simulink model "Encoder_reader_simulink"  (R2025a)
settings: Solver=FixedStepAuto  StartTime=0.0  StopTime=100  FixedStep=0.1  RelTol=1e-3  EnableMultiTasking=on
libraries: stm32f4xxblockslib x8, stm32g4xxblockslib x6
settings Model: STM32="{\"EncoderBlockForG4\":[{\"ID\":\"untitled:1\"},{\"ID\":\"Lab3_Encoder:1\"},{\"ID\":\"Encoder_reader_simulink:1\"},{\"ID\":\"Encoder_reader_simulink:35\"},{\"ID\":\"Encoder_reader_simulink:46\"},{\"ID\":\"Encoder_reader_simulink:93\"},{\"ID\":\"Encoder_reader_simulink:94\"},{\"ID\":\"Encoder_reader_simulink:95\"}],\"DigitalPortRead\":[{\"ID\":\"Encoder_reader_simulink:20\"},{\"ID\":\"Encoder_reader_simulink:21\"},{\"ID\":\"Encoder_reader_simulink:25\"},{\"ID\":\"Encoder_reader_simulink:32\"},{\"ID\":\"Encoder_reader_simulink:43\"},{\"ID\":\"Encoder_reader_simulink:90\"},{\"ID\":\"Encoder_reader_simulink:91\"},{\"ID\":\"Encoder_reader_simulink:92\"}]}"  Creator=User  LastModifiedBy=hp
settings OptimizationCC: DefaultParameterBehavior=Inlined  EnhancedBackFolding=on  PassReuseOutputArgsAs=Individual arguments  ZeroExternalMemoryAtStartup=off  ZeroInternalMemoryAtStartup=off  MaxStackSize=512  OptimizeBlockOrder=speed  DifferentSizesBufferReuse=on  OptimizationCustomize=off  EfficientTunableParamExpr=on
settings DebuggingCC: ParameterTunabilityLossMsg=error
settings HardwareCC: ProdBitPerPointer=32.0  ProdBitPerSizeT=32.0  ProdBitPerPtrDiffT=32.0  ProdLargestAtomicInteger=Long  ProdLargestAtomicFloat=Double  ProdWordSize=32.0  ProdLongLongMode=on  ProdHWDeviceType=ARM Compatible->ARM Cortex-M
settings SFSimCC: MATLABDynamicMemAlloc=off
settings RTWCC: SystemTargetFile=ert.tlc  HardwareBoard=STM32G4xx Based  TemplateMakefile=ert_default_tmf  Toolchain=GNU Tools for ARM Embedded Processors  Description=Embedded Coder
settings CodeAppCC: ForceParamTrailComments=on  IgnoreCustomStorageClasses=off  OperatorAnnotations=on  SimulinkDataObjDesc=on  SFDataObjDesc=on  InsertBlockDesc=on
settings ERTTargetCC: ExtModeTransport=3.0  ExtModeStaticAllocSize=2048.0  TargetLangStandard=C99 (ISO)  CodeReplacementLibrary=ARM Cortex-M  SupportContinuousTime=on

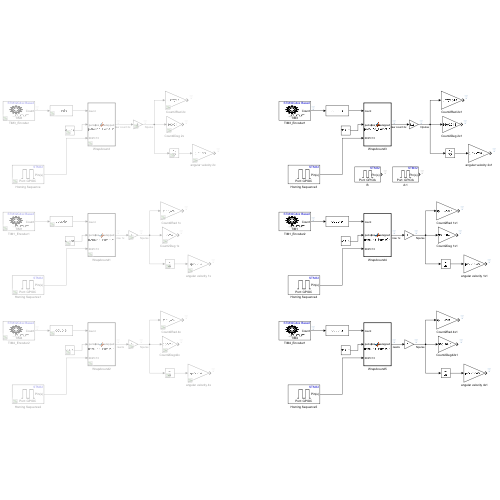
[thumbnail: Simulink's stored preview of the top-level diagram]
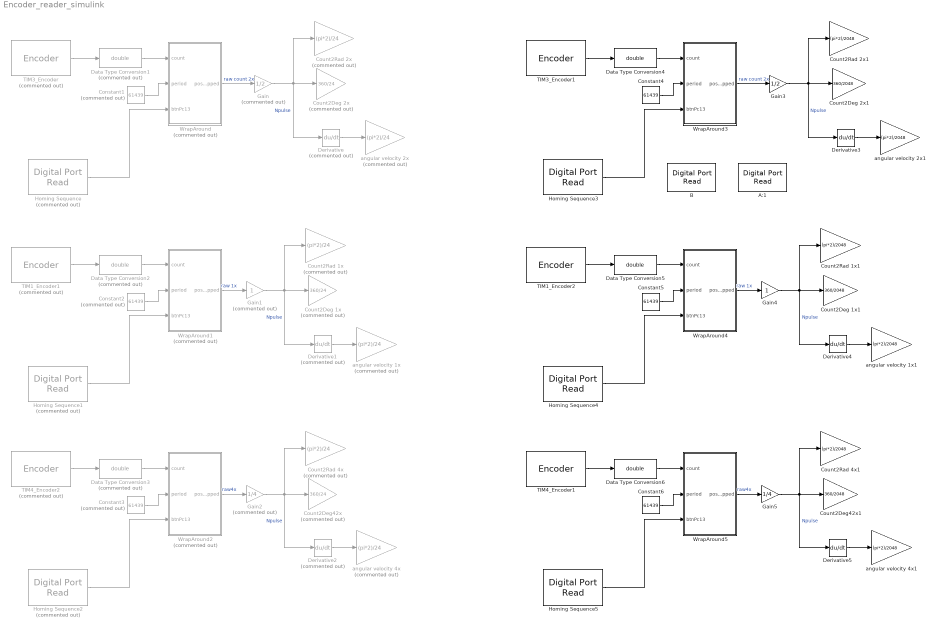
== system Encoder_reader_simulink ==
  A:1 : stm32f4xxblockslib/Digital Port Read  PortName=GPIOA  PinNumber=[4]  ReadOperation=on  IOAsArray=on  SampleTime=-1  EnableSimPort=off  hoistedMaskSrc=ECSoC/ECSimCodegen/Digital Port Read
      settings: LibrarySourceBlock=stm32g4xxblockslib/Digital Port Read
  B : stm32f4xxblockslib/Digital Port Read  PortName=GPIOA  PinNumber=[6]  ReadOperation=on  IOAsArray=on  SampleTime=-1  EnableSimPort=off  hoistedMaskSrc=ECSoC/ECSimCodegen/Digital Port Read
      settings: LibrarySourceBlock=stm32g4xxblockslib/Digital Port Read
  Constant1 : Constant  Commented=on  Value=61439
  Constant2 : Constant  Commented=on  Value=61439
  Constant3 : Constant  Commented=on  Value=61439
  Constant4 : Constant  Value=61439
  Constant5 : Constant  Value=61439
  Constant6 : Constant  Value=61439
  Count2Deg 1x : Gain  Commented=on  Gain=360/24
  Count2Deg 1x1 : Gain  Gain=360/2048
  Count2Deg 2x : Gain  Commented=on  Gain=360/24
  Count2Deg 2x1 : Gain  Gain=360/2048
  Count2Deg42x : Gain  Commented=on  Gain=360/24
  Count2Deg42x1 : Gain  Gain=360/2048
  Count2Rad 1x : Gain  Commented=on  Gain=(pi*2)/24
  Count2Rad 1x1 : Gain  Gain=(pi*2)/2048
  Count2Rad 2x : Gain  Commented=on  Gain=(pi*2)/24
  Count2Rad 2x1 : Gain  Gain=(pi*2)/2048
  Count2Rad 4x : Gain  Commented=on  Gain=(pi*2)/24
  Count2Rad 4x1 : Gain  Gain=(pi*2)/2048
  Data Type Conversion1 : DataTypeConversion  Commented=on  OutDataTypeStr=double  SaturateOnIntegerOverflow=off  RndMeth=Floor
  Data Type Conversion2 : DataTypeConversion  Commented=on  OutDataTypeStr=double  SaturateOnIntegerOverflow=off  RndMeth=Floor
  Data Type Conversion3 : DataTypeConversion  Commented=on  OutDataTypeStr=double  SaturateOnIntegerOverflow=off  RndMeth=Floor
  Data Type Conversion4 : DataTypeConversion  OutDataTypeStr=double  SaturateOnIntegerOverflow=off  RndMeth=Floor
  Data Type Conversion5 : DataTypeConversion  OutDataTypeStr=double  SaturateOnIntegerOverflow=off  RndMeth=Floor
  Data Type Conversion6 : DataTypeConversion  OutDataTypeStr=double  SaturateOnIntegerOverflow=off  RndMeth=Floor
  Derivative : Derivative  Commented=on
  Derivative1 : Derivative  Commented=on
  Derivative2 : Derivative  Commented=on
  Derivative3 : Derivative
  Derivative4 : Derivative
  Derivative5 : Derivative
  Gain : Gain  Commented=on  Gain=1/2
  Gain1 : Gain  Commented=on
  Gain2 : Gain  Commented=on  Gain=1/4
  Gain3 : Gain  Gain=1/2
  Gain4 : Gain
  Gain5 : Gain  Gain=1/4
  Homing Sequence : stm32f4xxblockslib/Digital Port Read  Commented=on  PortName=GPIOC  PinNumber=[13]  ReadOperation=on  IOAsArray=on  SampleTime=-1  EnableSimPort=off  hoistedMaskSrc=ECSoC/ECSimCodegen/Digital Port Read
      settings: LibrarySourceBlock=stm32g4xxblockslib/Digital Port Read
  Homing Sequence1 : stm32f4xxblockslib/Digital Port Read  Commented=on  PortName=GPIOC  PinNumber=[13]  ReadOperation=on  IOAsArray=on  SampleTime=-1  EnableSimPort=off  hoistedMaskSrc=ECSoC/ECSimCodegen/Digital Port Read
      settings: LibrarySourceBlock=stm32g4xxblockslib/Digital Port Read
  Homing Sequence2 : stm32f4xxblockslib/Digital Port Read  Commented=on  PortName=GPIOC  PinNumber=[13]  ReadOperation=on  IOAsArray=on  SampleTime=-1  EnableSimPort=off  hoistedMaskSrc=ECSoC/ECSimCodegen/Digital Port Read
      settings: LibrarySourceBlock=stm32g4xxblockslib/Digital Port Read
  Homing Sequence3 : stm32f4xxblockslib/Digital Port Read  PortName=GPIOC  PinNumber=[13]  ReadOperation=on  IOAsArray=on  SampleTime=-1  EnableSimPort=off  hoistedMaskSrc=ECSoC/ECSimCodegen/Digital Port Read
      settings: LibrarySourceBlock=stm32g4xxblockslib/Digital Port Read
  Homing Sequence4 : stm32f4xxblockslib/Digital Port Read  PortName=GPIOC  PinNumber=[13]  ReadOperation=on  IOAsArray=on  SampleTime=-1  EnableSimPort=off  hoistedMaskSrc=ECSoC/ECSimCodegen/Digital Port Read
      settings: LibrarySourceBlock=stm32g4xxblockslib/Digital Port Read
  Homing Sequence5 : stm32f4xxblockslib/Digital Port Read  PortName=GPIOC  PinNumber=[13]  ReadOperation=on  IOAsArray=on  SampleTime=-1  EnableSimPort=off  hoistedMaskSrc=ECSoC/ECSimCodegen/Digital Port Read
      settings: LibrarySourceBlock=stm32g4xxblockslib/Digital Port Read
  TIM1_Encoder1 : stm32g4xxblockslib/Encoder  Commented=on  TimerModule=TIM1  EnableResetInput=off  OutputCountAfterFirstIndex=off  OutputValidIndex=off  OutputDirection=off  OutputStatus=off  SampleTime=-1
  TIM1_Encoder2 : stm32g4xxblockslib/Encoder  TimerModule=TIM1  EnableResetInput=off  OutputCountAfterFirstIndex=off  OutputValidIndex=off  OutputDirection=off  OutputStatus=off  SampleTime=-1
  TIM3_Encoder : stm32g4xxblockslib/Encoder  Commented=on  TimerModule=TIM3  EnableResetInput=off  OutputCountAfterFirstIndex=off  OutputValidIndex=off  OutputDirection=off  OutputStatus=off  SampleTime=-1
  TIM3_Encoder1 : stm32g4xxblockslib/Encoder  TimerModule=TIM3  EnableResetInput=off  OutputCountAfterFirstIndex=off  OutputValidIndex=off  OutputDirection=off  OutputStatus=off  SampleTime=-1
  TIM4_Encoder1 : stm32g4xxblockslib/Encoder  TimerModule=TIM4  EnableResetInput=off  OutputCountAfterFirstIndex=off  OutputValidIndex=off  OutputDirection=off  OutputStatus=off  SampleTime=-1
  TIM4_Encoder2 : stm32g4xxblockslib/Encoder  Commented=on  TimerModule=TIM4  EnableResetInput=off  OutputCountAfterFirstIndex=off  OutputValidIndex=off  OutputDirection=off  OutputStatus=off  SampleTime=-1
  WrapAround : MATLAB Function  Commented=on  TreatAsAtomicUnit=on
  WrapAround1 : MATLAB Function  Commented=on  TreatAsAtomicUnit=on
  WrapAround2 : MATLAB Function  Commented=on  TreatAsAtomicUnit=on
  WrapAround3 : MATLAB Function  TreatAsAtomicUnit=on
  WrapAround4 : MATLAB Function  TreatAsAtomicUnit=on
  WrapAround5 : MATLAB Function  TreatAsAtomicUnit=on
  angular velocity 1x : Gain  Commented=on  Gain=(pi*2)/24
  angular velocity 1x1 : Gain  Gain=(pi*2)/2048
  angular velocity 2x : Gain  Commented=on  Gain=(pi*2)/24
  angular velocity 2x1 : Gain  Gain=(pi*2)/2048
  angular velocity 4x : Gain  Commented=on  Gain=(pi*2)/24
  angular velocity 4x1 : Gain  Gain=(pi*2)/2048
  wires:
  TIM3_Encoder/1 -> Data Type Conversion1/1
  Data Type Conversion1/1 -> WrapAround/1(count)
  WrapAround/1(pos_unwrapped) -> Gain/1  "raw count 2x"
  Constant1/1 -> WrapAround/2(period)
  Homing Sequence/1 -> WrapAround/3(btnPc13)
  Homing Sequence1/1 -> WrapAround1/3(btnPc13)
  WrapAround1/1(pos_unwrapped) -> Gain1/1  "raw 1x"
  Data Type Conversion2/1 -> WrapAround1/1(count)
  TIM1_Encoder1/1 -> Data Type Conversion2/1
  Constant2/1 -> WrapAround1/2(period)
  Homing Sequence2/1 -> WrapAround2/3(btnPc13)
  WrapAround2/1(pos_unwrapped) -> Gain2/1  "raw4x"
  Data Type Conversion3/1 -> WrapAround2/1(count)
  TIM4_Encoder2/1 -> Data Type Conversion3/1
  Constant3/1 -> WrapAround2/2(period)
  Gain/1 -> Derivative/1, Count2Deg 2x/1, Count2Rad 2x/1  "Npulse"
  Derivative/1 -> angular velocity 2x/1
  Derivative1/1 -> angular velocity 1x/1
  Gain1/1 -> Derivative1/1, Count2Deg 1x/1, Count2Rad 1x/1  "Npulse"
  Gain2/1 -> Derivative2/1, Count2Deg42x/1, Count2Rad 4x/1  "Npulse"
  Derivative2/1 -> angular velocity 4x/1
  WrapAround5/1(pos_unwrapped) -> Gain5/1  "raw4x"
  Derivative5/1 -> angular velocity 4x1/1
  Gain5/1 -> Derivative5/1, Count2Deg42x1/1, Count2Rad 4x1/1  "Npulse"
  Data Type Conversion5/1 -> WrapAround4/1(count)
  Homing Sequence4/1 -> WrapAround4/3(btnPc13)
  TIM1_Encoder2/1 -> Data Type Conversion5/1
  Derivative3/1 -> angular velocity 2x1/1
  Gain3/1 -> Derivative3/1, Count2Deg 2x1/1, Count2Rad 2x1/1  "Npulse"
  Constant6/1 -> WrapAround5/2(period)
  TIM4_Encoder1/1 -> Data Type Conversion6/1
  WrapAround3/1(pos_unwrapped) -> Gain3/1  "raw count 2x"
  Data Type Conversion6/1 -> WrapAround5/1(count)
  Derivative4/1 -> angular velocity 1x1/1
  Homing Sequence3/1 -> WrapAround3/3(btnPc13)
  Data Type Conversion4/1 -> WrapAround3/1(count)
  TIM3_Encoder1/1 -> Data Type Conversion4/1
  Constant5/1 -> WrapAround4/2(period)
  WrapAround4/1(pos_unwrapped) -> Gain4/1  "raw 1x"
  Homing Sequence5/1 -> WrapAround5/3(btnPc13)
  Gain4/1 -> Derivative4/1, Count2Deg 1x1/1, Count2Rad 1x1/1  "Npulse"
  Constant4/1 -> WrapAround3/2(period)

== matlab function Encoder_reader_simulink/WrapAround1 ==
  data: count input; pos_unwrapped output; period input; btnPc13 input
function pos_unwrapped = WrapAround_HomeOnPA5(count, period, btnPc13)
% WrapAround_HomeOnPA5
% - แก้ overflow ของ encoder counter และสะสมตำแหน่งต่อเนื่อง
% - เมื่อ "ปุ่ม PA5" ถูกกด (ขอบขาขึ้นหลังดีบาวน์) ให้รีเซ็ต pos_unwrapped = 0
%
% Inputs
%   count   : ค่าจาก TIMx encoder (0..period)
%   period  : ค่าขอบบนของเคาน์เตอร์ (เช่น 61439) → modulo = period+1
%   btnPc13  : 1 = ปุ่มถูกกด, 0 = ไม่กด (ถ้าเป็น active-low ให้ Invert มาก่อน)
%
% Output
%   pos_unwrapped : ตำแหน่งสะสมแบบต่อเนื่อง (รีเซ็ตเป็น 0 ตอนโฮม)

% ---------- สถานะภายใน ----------
persistent prevCount pos         % สำหรับแก้ wrap และสะสมตำแหน่ง
persistent stableBtn prevStable  % สำหรับดีบาวน์ + ตรวจขอบ
persistent cnt                   % ตัวนับดีบาวน์

if isempty(prevCount)
    prevCount   = double(count);
    pos         = 0.0;
    stableBtn   = false;   % สถานะปุ่มหลังดีบาวน์
    prevStable  = false;   % สถานะปุ่มดีบาวน์ย้อนหลัง 1 สเต็ป
    cnt         = uint16(0);
end

% ---------- แก้ wrap-around ----------
M    = double(period) + 1.0;     % โมดูลัสจริง
half = floor(M/2.0);
d = double(count) - prevCount;
if d >  half
    d = d - M;
elseif d < -half
    d = d + M;
end
pos = pos + d;
prevCount = double(count);

% ---------- ดีบาวน์ปุ่ม (แบบนับตัวอย่างติดกัน) ----------
% ปรับจำนวนตัวอย่างที่ต้องคงที่ก่อนยอมรับการเปลี่ยนสถานะ (N)
N = uint16(5);  % = 5 sample. ถ้า Ts = 1 ms → ~5 ms debounce

raw = (btnPc13 ~= 0);      % ให้เป็น boolean
if raw == stableBtn
    % ไม่มีแนวโน้มเปลี่ยนสถานะ → รีเซ็ตตัวนับ
    cnt = uint16(0);
else
    % มีแนวโน้มเปลี่ยน → นับต่อเนื่องจนถึง N แล้วค่อยสลับสถานะ
    if cnt < N
        cnt = cnt + 1;
    end
    if cnt >= N
        stableBtn = raw;
        cnt = uint16(0);
    end
end

% ---------- ตรวจขอบขาขึ้นหลังดีบาวน์ ----------
rising = (stableBtn == true) && (prevStable == false);
prevStable = stableBtn;

% ---------- รีเซ็ตตำแหน่งเมื่อกด ----------
if rising
    pos = 0.0;     % โฮม: ตั้งค่า pos_unwrapped = 0
end

% ---------- เอาต์พุต ----------
pos_unwrapped = -pos;
end

== matlab function Encoder_reader_simulink/WrapAround ==
  data: count input; pos_unwrapped output; period input; btnPc13 input
function pos_unwrapped=WrapAround_HomeOnPA5(count,period,btnPc13)
%Inputs:
%count   : ค่าจากตัวนับของ TIMx encoder
%period  : ค่าขอบบนของเคาน์เตอร์ (61439) → โมดูลัส = period + 1
%btnPc13 : สัญญาณปุ่ม 1 = กด, 0 = ไม่กด เพื่อ set home
%Output:
%pos_unwrapped : ตำแหน่งสะสมแบบต่อเนื่อง (รีเซ็ตเป็นศูนย์เมื่อโฮม)

persistent prevCount pos
persistent stableBtn prevStable
persistent cnt

if isempty(prevCount)
    % ตรวจว่าฟังก์ชันเพิ่งเริ่มทำงาน (ยังไม่มีค่าเก่า)
    prevCount=double(count);     % ตั้งค่า count เริ่มต้น
    pos=0.0;                     % เริ่มตำแหน่งที่ 0
    stableBtn=false;             % สถานะปุ่มเริ่มต้น = ไม่กด
    prevStable=false;            % สถานะก่อนหน้าเริ่มต้น = ไม่กด
    cnt=uint16(0);               % ตัวนับดีบาวน์เริ่มต้น = 0
end

M=double(period)+1.0;            % โมดูลัสจริงของเคาน์เตอร์ (เช่น 61439+1=61440)
half=floor(M/2.0);               % ครึ่งหนึ่งของโมดูลัส ใช้สำหรับตรวจการ overflow
d=double(count)-prevCount;       % คำนวณความต่างของ count ระหว่างรอบนี้กับรอบก่อน

if d>half
    d=d-M;                       % ถ้าค่ากระโดดบวกมากเกินครึ่ง → ถือว่า wrap จากสูงสุดไปต่ำสุด
elseif d<-half
    d=d+M;                       % ถ้าค่ากระโดดลบมากเกินครึ่ง → ถือว่า wrap จากต่ำสุดไปสูงสุด
end

pos=pos+d;                       % สะสมตำแหน่งแบบต่อเนื่อง (รวมระยะที่เปลี่ยน)
prevCount=double(count);         % เก็บค่า count ปัจจุบันไว้เป็นค่าเดิมสำหรับรอบถัดไป

%---------------- HOMING SEQUENCE ----------------%
N=uint16(5);                     % จำนวน sample ที่ใช้ดีบาวน์ปุ่ม (5 sample → ~5 ms)
raw=(btnPc13~=0);                % อ่านค่าปุ่ม → true ถ้ากด (แปลงเป็น boolean)

if raw==stableBtn
    cnt=uint16(0);               % ถ้าสถานะปุ่มไม่เปลี่ยน → รีเซ็ตตัวนับดีบาวน์
else
    if cnt<N
        cnt=cnt+1;               % ถ้ากำลังเปลี่ยนสถานะ → เพิ่มตัวนับ
    end
    if cnt>=N
        stableBtn=raw;           % ถ้าค่าคงที่ครบ N sample → ยอมรับสถานะใหม่
        cnt=uint16(0);           % รีเซ็ตตัวนับหลังยืนยันสถานะใหม่
    end
end

rising=(stableBtn==true)&&(prevStable==false);
% ตรวจขอบขาขึ้น (จากไม่กด → กด)

prevStable=stableBtn;            % เก็บสถานะปุ่มไว้เป็นค่าก่อนหน้าในรอบถัดไป

if rising
    pos=0.0;                     % ถ้ามีขอบขาขึ้น → รีเซ็ตตำแหน่ง = 0 (Home)
end

pos_unwrapped=-pos;              % สัญญาณเอาต์พุต (กลับขั้วทิศทาง)
end

== matlab function Encoder_reader_simulink/WrapAround2 ==
  data: count input; pos_unwrapped output; period input; btnPc13 input
function pos_unwrapped = WrapAround_HomeOnPA5(count, period, btnPc13)
% WrapAround_HomeOnPA5
% - แก้ overflow ของ encoder counter และสะสมตำแหน่งต่อเนื่อง
% - เมื่อ "ปุ่ม PA5" ถูกกด (ขอบขาขึ้นหลังดีบาวน์) ให้รีเซ็ต pos_unwrapped = 0
%
% Inputs
%   count   : ค่าจาก TIMx encoder (0..period)
%   period  : ค่าขอบบนของเคาน์เตอร์ (เช่น 61439) → modulo = period+1
%   btnPc13  : 1 = ปุ่มถูกกด, 0 = ไม่กด (ถ้าเป็น active-low ให้ Invert มาก่อน)
%
% Output
%   pos_unwrapped : ตำแหน่งสะสมแบบต่อเนื่อง (รีเซ็ตเป็น 0 ตอนโฮม)

% ---------- สถานะภายใน ----------
persistent prevCount pos         % สำหรับแก้ wrap และสะสมตำแหน่ง
persistent stableBtn prevStable  % สำหรับดีบาวน์ + ตรวจขอบ
persistent cnt                   % ตัวนับดีบาวน์

if isempty(prevCount)
    prevCount   = double(count);
    pos         = 0.0;
    stableBtn   = false;   % สถานะปุ่มหลังดีบาวน์
    prevStable  = false;   % สถานะปุ่มดีบาวน์ย้อนหลัง 1 สเต็ป
    cnt         = uint16(0);
end

% ---------- แก้ wrap-around ----------
M    = double(period) + 1.0;     % โมดูลัสจริง
half = floor(M/2.0);
d = double(count) - prevCount;
if d >  half
    d = d - M;
elseif d < -half
    d = d + M;
end
pos = pos + d;
prevCount = double(count);

% ---------- ดีบาวน์ปุ่ม (แบบนับตัวอย่างติดกัน) ----------
% ปรับจำนวนตัวอย่างที่ต้องคงที่ก่อนยอมรับการเปลี่ยนสถานะ (N)
N = uint16(5);  % = 5 sample. ถ้า Ts = 1 ms → ~5 ms debounce

raw = (btnPc13 ~= 0);      % ให้เป็น boolean
if raw == stableBtn
    % ไม่มีแนวโน้มเปลี่ยนสถานะ → รีเซ็ตตัวนับ
    cnt = uint16(0);
else
    % มีแนวโน้มเปลี่ยน → นับต่อเนื่องจนถึง N แล้วค่อยสลับสถานะ
    if cnt < N
        cnt = cnt + 1;
    end
    if cnt >= N
        stableBtn = raw;
        cnt = uint16(0);
    end
end

% ---------- ตรวจขอบขาขึ้นหลังดีบาวน์ ----------
rising = (stableBtn == true) && (prevStable == false);
prevStable = stableBtn;

% ---------- รีเซ็ตตำแหน่งเมื่อกด ----------
if rising
    pos = 0.0;     % โฮม: ตั้งค่า pos_unwrapped = 0
end

% ---------- เอาต์พุต ----------
pos_unwrapped = -pos;
end

== matlab function Encoder_reader_simulink/WrapAround3 ==
  data: count input; pos_unwrapped output; period input; btnPc13 input
function pos_unwrapped = WrapAround_HomeOnPA5(count, period, btnPc13)
persistent prevCount pos         % สำหรับแก้ wrap และสะสมตำแหน่ง
persistent stableBtn prevStable  % สำหรับดีบาวน์ + ตรวจขอบ
persistent cnt                   % ตัวนับดีบาวน์

if isempty(prevCount)
    prevCount   = double(count);
    pos         = 0.0;
    stableBtn   = false;   % สถานะปุ่มหลังดีบาวน์
    prevStable  = false;   % สถานะปุ่มดีบาวน์ย้อนหลัง 1 สเต็ป
    cnt         = uint16(0);
end
M    = double(period) + 1.0;     % โมดูลัสจริง
half = floor(M/2.0);
d = double(count) - prevCount;
if d >  half
    d = d - M;
elseif d < -half
    d = d + M;
end
pos = pos + d;
prevCount = double(count);
N = uint16(5);  % = 5 sample. ถ้า Ts = 1 ms → ~5 ms debounce

raw = (btnPc13 ~= 0);      % ให้เป็น boolean
if raw == stableBtn
    cnt = uint16(0);
else
    if cnt < N
        cnt = cnt + 1;
    end
    if cnt >= N
        stableBtn = raw;
        cnt = uint16(0);
    end
end
rising = (stableBtn == true) && (prevStable == false);
prevStable = stableBtn;

if rising
    pos = 0.0;     
end
pos_unwrapped = -pos;
end

== matlab function Encoder_reader_simulink/WrapAround4 ==
  data: count input; pos_unwrapped output; period input; btnPc13 input
function pos_unwrapped = WrapAround_HomeOnPA5(count, period, btnPc13)
% WrapAround_HomeOnPA5
% - แก้ overflow ของ encoder counter และสะสมตำแหน่งต่อเนื่อง
% - เมื่อ "ปุ่ม PA5" ถูกกด (ขอบขาขึ้นหลังดีบาวน์) ให้รีเซ็ต pos_unwrapped = 0
%
% Inputs
%   count   : ค่าจาก TIMx encoder (0..period)
%   period  : ค่าขอบบนของเคาน์เตอร์ (เช่น 61439) → modulo = period+1
%   btnPc13  : 1 = ปุ่มถูกกด, 0 = ไม่กด (ถ้าเป็น active-low ให้ Invert มาก่อน)
%
% Output
%   pos_unwrapped : ตำแหน่งสะสมแบบต่อเนื่อง (รีเซ็ตเป็น 0 ตอนโฮม)

% ---------- สถานะภายใน ----------
persistent prevCount pos         % สำหรับแก้ wrap และสะสมตำแหน่ง
persistent stableBtn prevStable  % สำหรับดีบาวน์ + ตรวจขอบ
persistent cnt                   % ตัวนับดีบาวน์

if isempty(prevCount)
    prevCount   = double(count);
    pos         = 0.0;
    stableBtn   = false;   % สถานะปุ่มหลังดีบาวน์
    prevStable  = false;   % สถานะปุ่มดีบาวน์ย้อนหลัง 1 สเต็ป
    cnt         = uint16(0);
end

% ---------- แก้ wrap-around ----------
M    = double(period) + 1.0;     % โมดูลัสจริง
half = floor(M/2.0);
d = double(count) - prevCount;
if d >  half
    d = d - M;
elseif d < -half
    d = d + M;
end
pos = pos + d;
prevCount = double(count);

% ---------- ดีบาวน์ปุ่ม (แบบนับตัวอย่างติดกัน) ----------
% ปรับจำนวนตัวอย่างที่ต้องคงที่ก่อนยอมรับการเปลี่ยนสถานะ (N)
N = uint16(5);  % = 5 sample. ถ้า Ts = 1 ms → ~5 ms debounce

raw = (btnPc13 ~= 0);      % ให้เป็น boolean
if raw == stableBtn
    % ไม่มีแนวโน้มเปลี่ยนสถานะ → รีเซ็ตตัวนับ
    cnt = uint16(0);
else
    % มีแนวโน้มเปลี่ยน → นับต่อเนื่องจนถึง N แล้วค่อยสลับสถานะ
    if cnt < N
        cnt = cnt + 1;
    end
    if cnt >= N
        stableBtn = raw;
        cnt = uint16(0);
    end
end

% ---------- ตรวจขอบขาขึ้นหลังดีบาวน์ ----------
rising = (stableBtn == true) && (prevStable == false);
prevStable = stableBtn;

% ---------- รีเซ็ตตำแหน่งเมื่อกด ----------
if rising
    pos = 0.0;     % โฮม: ตั้งค่า pos_unwrapped = 0
end

% ---------- เอาต์พุต ----------
pos_unwrapped = -pos;
end

== matlab function Encoder_reader_simulink/WrapAround5 ==
  data: count input; pos_unwrapped output; period input; btnPc13 input
function pos_unwrapped = WrapAround_HomeOnPA5(count, period, btnPc13)
% WrapAround_HomeOnPA5
% - แก้ overflow ของ encoder counter และสะสมตำแหน่งต่อเนื่อง
% - เมื่อ "ปุ่ม PA5" ถูกกด (ขอบขาขึ้นหลังดีบาวน์) ให้รีเซ็ต pos_unwrapped = 0
%
% Inputs
%   count   : ค่าจาก TIMx encoder (0..period)
%   period  : ค่าขอบบนของเคาน์เตอร์ (เช่น 61439) → modulo = period+1
%   btnPc13  : 1 = ปุ่มถูกกด, 0 = ไม่กด (ถ้าเป็น active-low ให้ Invert มาก่อน)
%
% Output
%   pos_unwrapped : ตำแหน่งสะสมแบบต่อเนื่อง (รีเซ็ตเป็น 0 ตอนโฮม)

% ---------- สถานะภายใน ----------
persistent prevCount pos         % สำหรับแก้ wrap และสะสมตำแหน่ง
persistent stableBtn prevStable  % สำหรับดีบาวน์ + ตรวจขอบ
persistent cnt                   % ตัวนับดีบาวน์

if isempty(prevCount)
    prevCount   = double(count);
    pos         = 0.0;
    stableBtn   = false;   % สถานะปุ่มหลังดีบาวน์
    prevStable  = false;   % สถานะปุ่มดีบาวน์ย้อนหลัง 1 สเต็ป
    cnt         = uint16(0);
end

% ---------- แก้ wrap-around ----------
M    = double(period) + 1.0;     % โมดูลัสจริง
half = floor(M/2.0);
d = double(count) - prevCount;
if d >  half
    d = d - M;
elseif d < -half
    d = d + M;
end
pos = pos + d;
prevCount = double(count);

% ---------- ดีบาวน์ปุ่ม (แบบนับตัวอย่างติดกัน) ----------
% ปรับจำนวนตัวอย่างที่ต้องคงที่ก่อนยอมรับการเปลี่ยนสถานะ (N)
N = uint16(5);  % = 5 sample. ถ้า Ts = 1 ms → ~5 ms debounce

raw = (btnPc13 ~= 0);      % ให้เป็น boolean
if raw == stableBtn
    % ไม่มีแนวโน้มเปลี่ยนสถานะ → รีเซ็ตตัวนับ
    cnt = uint16(0);
else
    % มีแนวโน้มเปลี่ยน → นับต่อเนื่องจนถึง N แล้วค่อยสลับสถานะ
    if cnt < N
        cnt = cnt + 1;
    end
    if cnt >= N
        stableBtn = raw;
        cnt = uint16(0);
    end
end

% ---------- ตรวจขอบขาขึ้นหลังดีบาวน์ ----------
rising = (stableBtn == true) && (prevStable == false);
prevStable = stableBtn;

% ---------- รีเซ็ตตำแหน่งเมื่อกด ----------
if rising
    pos = 0.0;     % โฮม: ตั้งค่า pos_unwrapped = 0
end

% ---------- เอาต์พุต ----------
pos_unwrapped = -pos;
end
